simulink model "Registri"  (R2018b)
settings: Solver=FixedStepAuto  StartTime=0.0  StopTime=20  RelTol=1e-3
settings Model: DataTypeOverride=Off  Creator=fabio  LastModifiedBy=fabio
settings DataIOCC: LimitDataPoints=on  SaveOutput=off  SaveTime=off
settings OptimizationCC: BlockReduction=off  ConditionallyExecuteInputs=off  DefaultParameterBehavior=Inlined  LifeSpan=inf
settings DebuggingCC: AlgebraicLoopMsg=error  SingleTaskRateTransMsg=error  AllowSymbolicDim=off  StrictBusMsg=ErrorOnBusTreatedAsVector  SFUnexpectedBacktrackingDiag=warning  SFNoUnconditionalDefaultTransitionDiag=warning  SFExecutionAtInitializationDiag=none
settings HardwareCC: ProdBitPerPointer=32  ProdBitPerSizeT=32  ProdBitPerPtrDiffT=32  ProdLargestAtomicFloat=None  ProdIntDivRoundTo=Undefined  ProdEndianess=Unspecified  ProdWordSize=32  ProdHWDeviceType=ASIC/FPGA->ASIC/FPGA  ProdEqTarget=off
settings SFSimCC: SimUseLocalCustomCode=off
settings RTWCC: RTWUseLocalCustomCode=off
settings CodeAppCC: StateflowObjectComments=on
settings GRTTargetCC: TargetLangStandard=C89/C90 (ANSI)  GeneratePreprocessorConditionals=Disable all
settings ConfigComp: CovScope=ReferencedModels  CovMetricSettings=dw  CovHtmlReporting=on  CovSaveCumulativeToWorkspaceVar=on  CovSaveSingleToWorkspaceVar=on  CovExternalEMLEnable=off  CovSFcnEnable=off

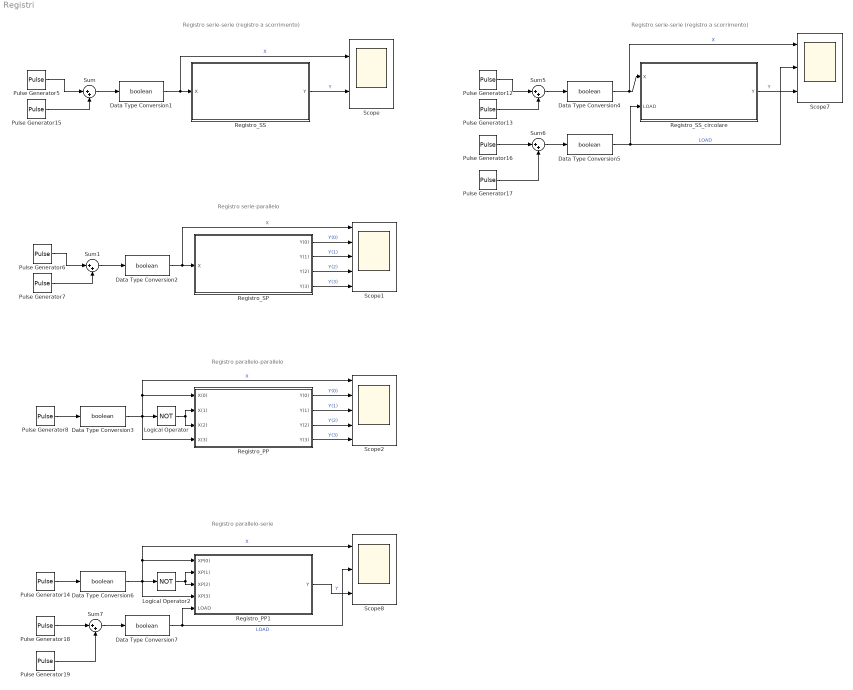
== system Registri ==
  note: Registro serie-serie (registro a scorrimento)
  note: Registro serie-parallelo
  note: Registro parallelo-parallelo
  note: Registro serie-serie (registro a scorrimento)
  note: Registro parallelo-serie
  Data Type Conversion{1..7} (7 alike) : DataTypeConversion  OutDataTypeStr=boolean
  Logical Operator : Logic  Operator=NOT  IconShape=distinctive  AllPortsSameDT=off  OutDataTypeStr=boolean
  Logical Operator2 : Logic  Operator=NOT  IconShape=distinctive  AllPortsSameDT=off  OutDataTypeStr=boolean
  Pulse Generator{5..6,12,16,18} (5 alike) : DiscretePulseGenerator  PulseType=Time based  Period=100  PhaseDelay=1
  Pulse Generator13 : DiscretePulseGenerator  PulseType=Time based  Period=100  PhaseDelay=6
  Pulse Generator14 : DiscretePulseGenerator  PulseType=Time based  Period=100  PulseWidth=5  PhaseDelay=1
  Pulse Generator15 : DiscretePulseGenerator  PulseType=Time based  Period=100  PhaseDelay=6
  Pulse Generator17 : DiscretePulseGenerator  PulseType=Time based  Period=100  PhaseDelay=13
  Pulse Generator19 : DiscretePulseGenerator  PulseType=Time based  Period=100  PhaseDelay=13
  Pulse Generator7 : DiscretePulseGenerator  PulseType=Time based  Period=100  PhaseDelay=6
  Pulse Generator8 : DiscretePulseGenerator  PulseType=Time based  Period=100  PulseWidth=5  PhaseDelay=1
  Registro_PP : Subsystem
  Registro_PP1 : Subsystem
  Registro_SP : Subsystem
  Registro_SS : Subsystem
  Registro_SS_circolare : Subsystem
  Scope : Scope  NumInputPorts=2
  Scope1 : Scope  NumInputPorts=5
  Scope2 : Scope  NumInputPorts=5
  Scope7 : Scope  NumInputPorts=3
  Scope8 : Scope  NumInputPorts=3
  Sum{,1,5..7} (5 alike) : Sum  Inputs=|++
  wires:
  Registro_SS/1(Y) -> Scope/2  "Y"
  Sum1/1 -> Data Type Conversion2/1
  Logical Operator/1 -> Registro_PP/3(X(2)), Registro_PP/2(X(1))
  Pulse Generator5/1 -> Sum/1
  Pulse Generator8/1 -> Data Type Conversion3/1
  Registro_PP/1(Y(0)) -> Scope2/2  "Y(0)"
  Registro_SP/1(Y(0)) -> Scope1/2  "Y(0)"
  Registro_SP/2(Y(1)) -> Scope1/3  "Y(1)"
  Registro_SP/3(Y(2)) -> Scope1/4  "Y(2)"
  Registro_SP/4(Y(3)) -> Scope1/5  "Y(3)"
  Registro_PP/2(Y(1)) -> Scope2/3  "Y(1)"
  Registro_PP/3(Y(2)) -> Scope2/4  "Y(2)"
  Registro_PP/4(Y(3)) -> Scope2/5  "Y(3)"
  Sum/1 -> Data Type Conversion1/1
  Pulse Generator15/1 -> Sum/2
  Pulse Generator6/1 -> Sum1/1
  Pulse Generator7/1 -> Sum1/2
  Data Type Conversion1/1 -> Scope/1, Registro_SS/1(X)  "X"
  Data Type Conversion2/1 -> Scope1/1, Registro_SP/1(X)  "X"
  Data Type Conversion3/1 -> Registro_PP/4(X(3)), Logical Operator/1, Scope2/1, Registro_PP/1(X(0))  "X"
  Pulse Generator12/1 -> Sum5/1
  Pulse Generator13/1 -> Sum5/2
  Sum5/1 -> Data Type Conversion4/1
  Data Type Conversion4/1 -> Scope7/1, Registro_SS_circolare/1(X)  "X"
  Registro_SS_circolare/1(Y) -> Scope7/3  "Y"
  Data Type Conversion5/1 -> Scope7/2, Registro_SS_circolare/2(LOAD)  "LOAD"
  Pulse Generator16/1 -> Sum6/1
  Sum6/1 -> Data Type Conversion5/1
  Pulse Generator17/1 -> Sum6/2
  Pulse Generator14/1 -> Data Type Conversion6/1
  Logical Operator2/1 -> Registro_PP1/3(XP(2)), Registro_PP1/2(XP(1))
  Data Type Conversion6/1 -> Registro_PP1/4(XP(3)), Logical Operator2/1, Scope8/1, Registro_PP1/1(XP(0))  "X"
  Registro_PP1/1(Y) -> Scope8/3  "Y"
  Sum7/1 -> Data Type Conversion7/1
  Pulse Generator18/1 -> Sum7/1
  Pulse Generator19/1 -> Sum7/2
  Data Type Conversion7/1 -> Scope8/2, Registro_PP1/5(LOAD)  "LOAD"

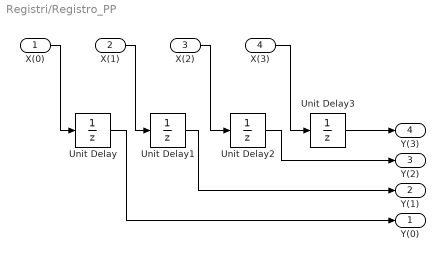
== system Registri/Registro_PP ==
  X(0) : Inport
  X(1) : Inport  Port=2
  X(2) : Inport  Port=3
  X(3) : Inport  Port=4
  Unit Delay{,1..3} (4 alike) : UnitDelay  SampleTime=-1
  Y(0) : Outport
  Y(1) : Outport  Port=2
  Y(2) : Outport  Port=3
  Y(3) : Outport  Port=4
  wires:
  Unit Delay1/1 -> Y(1)/1
  Unit Delay2/1 -> Y(2)/1
  Unit Delay/1 -> Y(0)/1
  Unit Delay3/1 -> Y(3)/1
  X(0)/1 -> Unit Delay/1
  X(3)/1 -> Unit Delay3/1
  X(2)/1 -> Unit Delay2/1
  X(1)/1 -> Unit Delay1/1

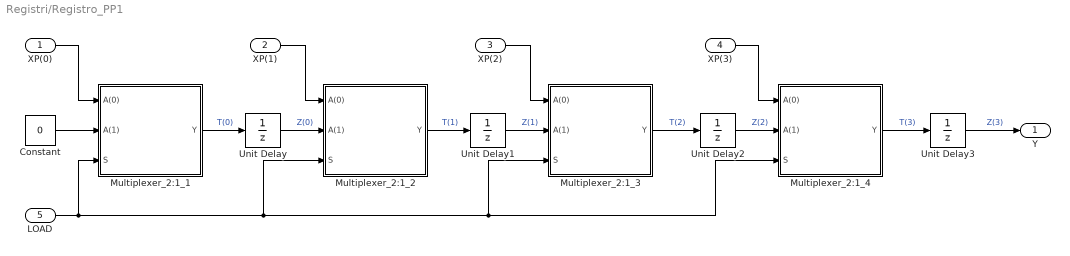
== system Registri/Registro_PP1 ==
  XP(0) : Inport
  XP(1) : Inport  Port=2
  XP(2) : Inport  Port=3
  XP(3) : Inport  Port=4
  LOAD : Inport  Port=5
  Constant : Constant  Value=0  OutDataTypeStr=boolean
  Multiplexer_2:1_1 : Subsystem
  Multiplexer_2:1_2 : Subsystem
  Multiplexer_2:1_3 : Subsystem
  Multiplexer_2:1_4 : Subsystem
  Unit Delay{,1..3} (4 alike) : UnitDelay  SampleTime=-1
  Y : Outport
  wires:
  XP(0)/1 -> Multiplexer_2:1_1/1(A(0))
  Multiplexer_2:1_1/1(Y) -> Unit Delay/1  "T(0)"
  XP(1)/1 -> Multiplexer_2:1_2/1(A(0))
  Unit Delay/1 -> Multiplexer_2:1_2/2(A(1))  "Z(0)"
  Constant/1 -> Multiplexer_2:1_1/2(A(1))
  Multiplexer_2:1_2/1(Y) -> Unit Delay1/1  "T(1)"
  Unit Delay1/1 -> Multiplexer_2:1_3/2(A(1))  "Z(1)"
  XP(2)/1 -> Multiplexer_2:1_3/1(A(0))
  Multiplexer_2:1_3/1(Y) -> Unit Delay2/1  "T(2)"
  Unit Delay2/1 -> Multiplexer_2:1_4/2(A(1))  "Z(2)"
  Multiplexer_2:1_4/1(Y) -> Unit Delay3/1  "T(3)"
  XP(3)/1 -> Multiplexer_2:1_4/1(A(0))
  Unit Delay3/1 -> Y/1  "Z(3)"
  LOAD/1 -> Multiplexer_2:1_2/3(S), Multiplexer_2:1_4/3(S), Multiplexer_2:1_3/3(S), Multiplexer_2:1_1/3(S)

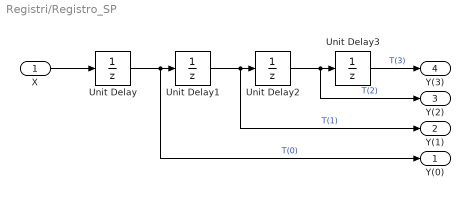
== system Registri/Registro_SP ==
  X : Inport
  Unit Delay{,1..3} (4 alike) : UnitDelay  SampleTime=-1
  Y(0) : Outport
  Y(1) : Outport  Port=2
  Y(2) : Outport  Port=3
  Y(3) : Outport  Port=4
  wires:
  Unit Delay1/1 -> Y(1)/1, Unit Delay2/1  "T(1)"
  Unit Delay2/1 -> Y(2)/1, Unit Delay3/1  "T(2)"
  Unit Delay/1 -> Y(0)/1, Unit Delay1/1  "T(0)"
  Unit Delay3/1 -> Y(3)/1  "T(3)"
  X/1 -> Unit Delay/1

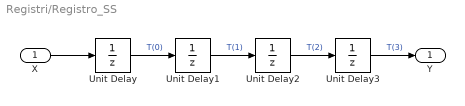
== system Registri/Registro_SS ==
  X : Inport
  Unit Delay{,1..3} (4 alike) : UnitDelay  SampleTime=-1
  Y : Outport
  wires:
  Unit Delay1/1 -> Unit Delay2/1  "T(1)"
  Unit Delay2/1 -> Unit Delay3/1  "T(2)"
  Unit Delay/1 -> Unit Delay1/1  "T(0)"
  Unit Delay3/1 -> Y/1  "T(3)"
  X/1 -> Unit Delay/1

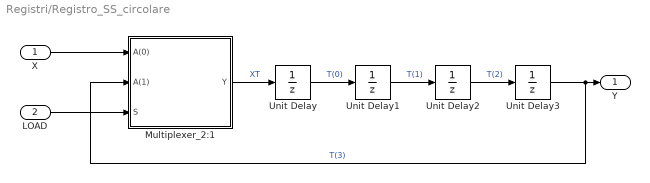
== system Registri/Registro_SS_circolare ==
  X : Inport
  LOAD : Inport  Port=2
  Multiplexer_2:1 : Subsystem
  Unit Delay{,1..3} (4 alike) : UnitDelay  SampleTime=-1
  Y : Outport
  wires:
  Unit Delay1/1 -> Unit Delay2/1  "T(1)"
  Unit Delay2/1 -> Unit Delay3/1  "T(2)"
  Unit Delay/1 -> Unit Delay1/1  "T(0)"
  Unit Delay3/1 -> Multiplexer_2:1/2(A(1)), Y/1  "T(3)"
  Multiplexer_2:1/1(Y) -> Unit Delay/1  "XT"
  X/1 -> Multiplexer_2:1/1(A(0))
  LOAD/1 -> Multiplexer_2:1/3(S)

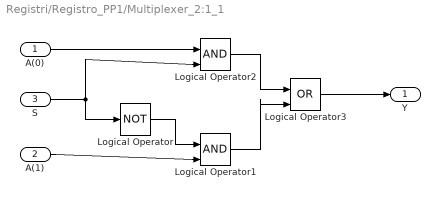
== system Registri/Registro_PP1/Multiplexer_2:1_1 ==
  A(0) : Inport
  A(1) : Inport  Port=2
  S : Inport  Port=3
  Logical Operator : Logic  Operator=NOT  IconShape=distinctive  AllPortsSameDT=off  OutDataTypeStr=boolean
  Logical Operator1 : Logic  IconShape=distinctive  AllPortsSameDT=off  OutDataTypeStr=boolean
  Logical Operator2 : Logic  IconShape=distinctive  AllPortsSameDT=off  OutDataTypeStr=boolean
  Logical Operator3 : Logic  Operator=OR  IconShape=distinctive  AllPortsSameDT=off  OutDataTypeStr=boolean
  Y : Outport
  wires:
  S/1 -> Logical Operator2/2, Logical Operator/1
  A(1)/1 -> Logical Operator1/2
  Logical Operator/1 -> Logical Operator1/1
  A(0)/1 -> Logical Operator2/1
  Logical Operator2/1 -> Logical Operator3/1
  Logical Operator1/1 -> Logical Operator3/2
  Logical Operator3/1 -> Y/1

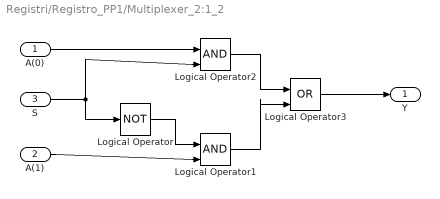
== system Registri/Registro_PP1/Multiplexer_2:1_2 ==
  A(0) : Inport
  A(1) : Inport  Port=2
  S : Inport  Port=3
  Logical Operator : Logic  Operator=NOT  IconShape=distinctive  AllPortsSameDT=off  OutDataTypeStr=boolean
  Logical Operator1 : Logic  IconShape=distinctive  AllPortsSameDT=off  OutDataTypeStr=boolean
  Logical Operator2 : Logic  IconShape=distinctive  AllPortsSameDT=off  OutDataTypeStr=boolean
  Logical Operator3 : Logic  Operator=OR  IconShape=distinctive  AllPortsSameDT=off  OutDataTypeStr=boolean
  Y : Outport
  wires:
  S/1 -> Logical Operator2/2, Logical Operator/1
  A(1)/1 -> Logical Operator1/2
  Logical Operator/1 -> Logical Operator1/1
  A(0)/1 -> Logical Operator2/1
  Logical Operator2/1 -> Logical Operator3/1
  Logical Operator1/1 -> Logical Operator3/2
  Logical Operator3/1 -> Y/1

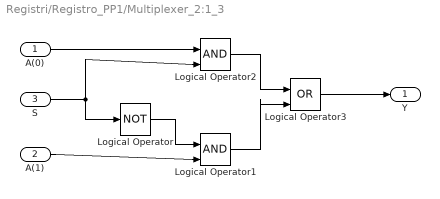
== system Registri/Registro_PP1/Multiplexer_2:1_3 ==
  A(0) : Inport
  A(1) : Inport  Port=2
  S : Inport  Port=3
  Logical Operator : Logic  Operator=NOT  IconShape=distinctive  AllPortsSameDT=off  OutDataTypeStr=boolean
  Logical Operator1 : Logic  IconShape=distinctive  AllPortsSameDT=off  OutDataTypeStr=boolean
  Logical Operator2 : Logic  IconShape=distinctive  AllPortsSameDT=off  OutDataTypeStr=boolean
  Logical Operator3 : Logic  Operator=OR  IconShape=distinctive  AllPortsSameDT=off  OutDataTypeStr=boolean
  Y : Outport
  wires:
  S/1 -> Logical Operator2/2, Logical Operator/1
  A(1)/1 -> Logical Operator1/2
  Logical Operator/1 -> Logical Operator1/1
  A(0)/1 -> Logical Operator2/1
  Logical Operator2/1 -> Logical Operator3/1
  Logical Operator1/1 -> Logical Operator3/2
  Logical Operator3/1 -> Y/1

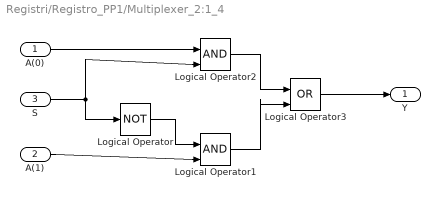
== system Registri/Registro_PP1/Multiplexer_2:1_4 ==
  A(0) : Inport
  A(1) : Inport  Port=2
  S : Inport  Port=3
  Logical Operator : Logic  Operator=NOT  IconShape=distinctive  AllPortsSameDT=off  OutDataTypeStr=boolean
  Logical Operator1 : Logic  IconShape=distinctive  AllPortsSameDT=off  OutDataTypeStr=boolean
  Logical Operator2 : Logic  IconShape=distinctive  AllPortsSameDT=off  OutDataTypeStr=boolean
  Logical Operator3 : Logic  Operator=OR  IconShape=distinctive  AllPortsSameDT=off  OutDataTypeStr=boolean
  Y : Outport
  wires:
  S/1 -> Logical Operator2/2, Logical Operator/1
  A(1)/1 -> Logical Operator1/2
  Logical Operator/1 -> Logical Operator1/1
  A(0)/1 -> Logical Operator2/1
  Logical Operator2/1 -> Logical Operator3/1
  Logical Operator1/1 -> Logical Operator3/2
  Logical Operator3/1 -> Y/1

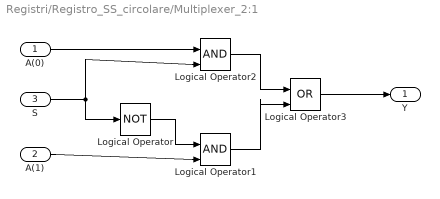
== system Registri/Registro_SS_circolare/Multiplexer_2:1 ==
  A(0) : Inport
  A(1) : Inport  Port=2
  S : Inport  Port=3
  Logical Operator : Logic  Operator=NOT  IconShape=distinctive  AllPortsSameDT=off  OutDataTypeStr=boolean
  Logical Operator1 : Logic  IconShape=distinctive  AllPortsSameDT=off  OutDataTypeStr=boolean
  Logical Operator2 : Logic  IconShape=distinctive  AllPortsSameDT=off  OutDataTypeStr=boolean
  Logical Operator3 : Logic  Operator=OR  IconShape=distinctive  AllPortsSameDT=off  OutDataTypeStr=boolean
  Y : Outport
  wires:
  S/1 -> Logical Operator2/2, Logical Operator/1
  A(1)/1 -> Logical Operator1/2
  Logical Operator/1 -> Logical Operator1/1
  A(0)/1 -> Logical Operator2/1
  Logical Operator2/1 -> Logical Operator3/1
  Logical Operator1/1 -> Logical Operator3/2
  Logical Operator3/1 -> Y/1
